simulink model "QPSK_mod_demod_Simulink_Block_Diagram"  (R2020b)
settings: Solver=VariableStepAuto  StartTime=0.0  StopTime=0.05  RelTol=1e-3
libraries: dspsrcs4 x4, simulink x3, dsparch4 x2, commseqgen3 x1, eeGeneralControl x1
settings Model: Creator=harshit  LastModifiedBy=Mohit Akhouri
settings SFSimCC: CustomCodeUndefinedFunction=UseInterfaceOnly

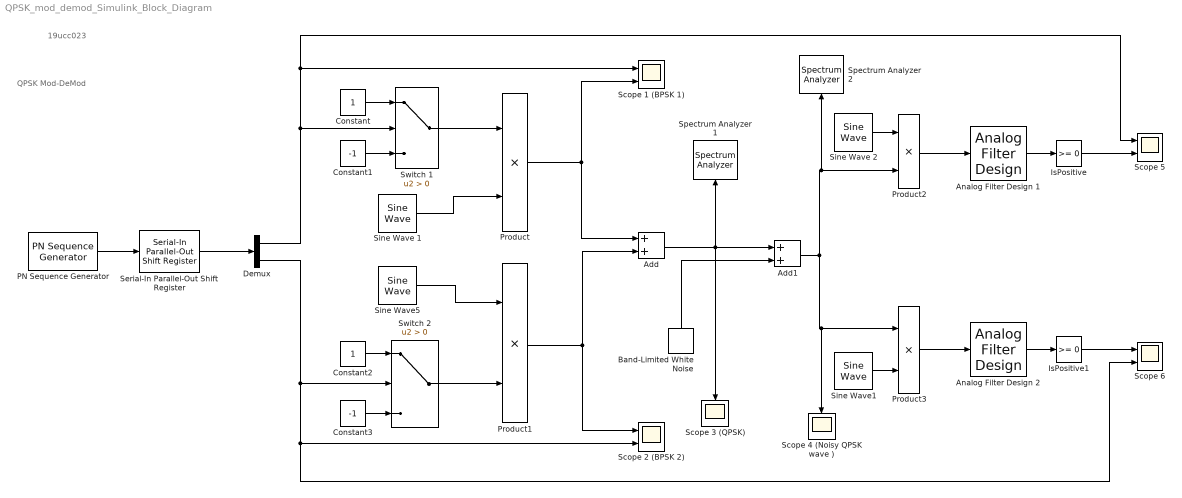
== system QPSK_mod_demod_Simulink_Block_Diagram ==
  note: QPSK Mod-DeMod
  note: 19ucc023
  Add : Sum
  Add1 : Sum
  Analog Filter Design 1 : dsparch4/Analog Filter Design  method=Butterworth  filttype=Lowpass  N=8  Wlo=2*pi*2000  Whi=80  Rp=2  Rs=40
  Analog Filter Design 2 : dsparch4/Analog Filter Design  method=Butterworth  filttype=Lowpass  N=8  Wlo=2*pi*2000  Whi=80  Rp=2  Rs=40
  Band-Limited White Noise : simulink/Sources/Band-Limited White Noise  Cov=[0.00001]  Ts=0.001  seed=[23341]
  Constant : Constant
  Constant1 : Constant  Value=-1
  Constant2 : Constant
  Constant3 : Constant  Value=-1
  Demux : Demux  Outputs=2
  IsPositive : simulink/Logic and Bit Operations/Compare To Zero  relop=>=  OutDataTypeStr=boolean
  IsPositive1 : simulink/Logic and Bit Operations/Compare To Zero  relop=>=  OutDataTypeStr=boolean
  PN Sequence Generator : commseqgen3/PN Sequence Generator  poly='z^6 + z^3 + 1'  ini_sta=[0 0 0 0 0 1]  outBitMaskSource=Dialog parameter  shift=0  outVarSiz=off  maxOutSizeMode=Dialog parameter  maxOutSize=[10 1]  Ts=1  sampPerFrame=1  reset=off  bitPackedOutputs=off  outDataType=double  numPackedBits=8  bitPackDataSigned=off  bitPackedOutDType=double
      settings: SourceProductName=Communications Toolbox
  Product{,1..3} (4 alike) : Product
  Scope 1 (BPSK 1) : Scope  NumInputPorts=2
  Scope 2 (BPSK 2) : Scope  NumInputPorts=2
  Scope 3 (QPSK) : Scope
  Scope 4 (Noisy QPSK wave ) : Scope
  Scope 5 : Scope  NumInputPorts=2
  Scope 6 : Scope  NumInputPorts=2
  Serial-In Parallel-Out Shift Register : eeGeneralControl/Serial-In Parallel-Out Shift Register  N=2  IC=0  Ts=-1
      settings: SourceProductBaseCode=PS
  Sine Wave 1 : dspsrcs4/Sine Wave  Amplitude=1  Frequency=2*pi*1000  Phase=0  SampleMode=Discrete  OutComplex=Real  CompMethod=Trigonometric fcn  TableSize=Speed  SampleTime=1/1000  SamplesPerFrame=1  ResetState=Restart at time zero  OutputFrames=off  dataType=double  wordLen=16  udDataType=sfix(16)  fracBitsMode=Best precision  numFracBits=15  OutDataTypeStr=double  LastOutDataTypeStr=double
  Sine Wave 2 : dspsrcs4/Sine Wave  Amplitude=1  Frequency=2*pi*1000  Phase=0  SampleMode=Discrete  OutComplex=Real  CompMethod=Trigonometric fcn  TableSize=Speed  SampleTime=1/1000  SamplesPerFrame=1  ResetState=Restart at time zero  OutputFrames=off  dataType=double  wordLen=16  udDataType=sfix(16)  fracBitsMode=Best precision  numFracBits=15  OutDataTypeStr=double  LastOutDataTypeStr=double
  Sine Wave1 : dspsrcs4/Sine Wave  Amplitude=1  Frequency=2*pi*1000  Phase=pi/2  SampleMode=Discrete  OutComplex=Real  CompMethod=Trigonometric fcn  TableSize=Speed  SampleTime=1/1000  SamplesPerFrame=1  ResetState=Restart at time zero  OutputFrames=off  dataType=double  wordLen=16  udDataType=sfix(16)  fracBitsMode=Best precision  numFracBits=15  OutDataTypeStr=double  LastOutDataTypeStr=double
  Sine Wave5 : dspsrcs4/Sine Wave  Amplitude=1  Frequency=2*pi*1000  Phase=pi/2  SampleMode=Discrete  OutComplex=Real  CompMethod=Trigonometric fcn  TableSize=Speed  SampleTime=1/1000  SamplesPerFrame=1  ResetState=Restart at time zero  OutputFrames=off  dataType=double  wordLen=16  udDataType=sfix(16)  fracBitsMode=Best precision  numFracBits=15  OutDataTypeStr=double  LastOutDataTypeStr=double
  Spectrum Analyzer 1 : SpectrumAnalyzer
  Spectrum Analyzer 2 : SpectrumAnalyzer
  Switch 1 : Switch  Criteria=u2 > Threshold
  Switch 2 : Switch  Criteria=u2 > Threshold
  wires:
  Constant/1 -> Switch 1/1
  Constant1/1 -> Switch 1/3
  Constant2/1 -> Switch 2/1
  Constant3/1 -> Switch 2/3
  Switch 1/1 -> Product/1
  Switch 2/1 -> Product1/2
  Product/1 -> Add/1, Scope 1 (BPSK 1)/2
  Product1/1 -> Scope 2 (BPSK 2)/1, Add/2
  Add/1 -> Scope 3 (QPSK)/1, Spectrum Analyzer 1/1, Add1/1
  Band-Limited White Noise/1 -> Add1/2
  Add1/1 -> Product2/2, Spectrum Analyzer 2/1, Product3/1, Scope 4 (Noisy QPSK wave )/1
  Product2/1 -> Analog Filter Design 1/1
  Product3/1 -> Analog Filter Design 2/1
  Analog Filter Design 1/1 -> IsPositive/1
  Analog Filter Design 2/1 -> IsPositive1/1
  Sine Wave1/1 -> Product3/2
  Sine Wave 2/1 -> Product2/1
  IsPositive/1 -> Scope 5/2
  IsPositive1/1 -> Scope 6/1
  PN Sequence Generator/1 -> Serial-In Parallel-Out Shift Register/1
  Serial-In Parallel-Out Shift Register/1 -> Demux/1
  Demux/1 -> Scope 5/1, Scope 1 (BPSK 1)/1, Switch 1/2
  Demux/2 -> Switch 2/2, Scope 6/2, Scope 2 (BPSK 2)/2
  Sine Wave 1/1 -> Product/2
  Sine Wave5/1 -> Product1/1
